simulink model "punto3"  (R2017b)
settings: Solver=VariableStepAuto  StartTime=0.0  StopTime=.3  RelTol=1e-3
values from neighbouring files (symbols this model uses):
  T0 = 0.015    [Practica2Control3.m]
  Tcarga = 0.15    [Practica2Control3.m]
  Va = 100    [Practica2Control3.m]
undefined symbols (not defined in the file or in its folder): d1c, d1d, d2d, n1c, n1d, n2c, n2d
settings Model: Creator=Agustin  LastModifiedBy=Agustin

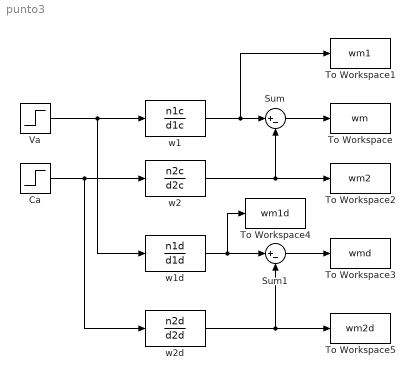
== system punto3 ==
  Ca : Step  Time=Tcarga  SampleTime=0
  Sum : Sum  Inputs=|+-
  Sum1 : Sum  Inputs=|+-
  To Workspace : ToWorkspace  VariableName=wm  SaveFormat=Timeseries  SampleTime=-1
  To Workspace1 : ToWorkspace  VariableName=wm1  SaveFormat=Timeseries  SampleTime=-1
  To Workspace2 : ToWorkspace  VariableName=wm2  SaveFormat=Timeseries  SampleTime=-1
  To Workspace3 : ToWorkspace  VariableName=wmd  SaveFormat=Timeseries  SampleTime=-1
  To Workspace4 : ToWorkspace  VariableName=wm1d  SaveFormat=Timeseries  SampleTime=-1
  To Workspace5 : ToWorkspace  VariableName=wm2d  SaveFormat=Timeseries  SampleTime=-1
  Va : Step  Time=0  After=Va  SampleTime=0
  w1 : TransferFcn  Numerator=n1c  Denominator=d1c
  w1d : DiscreteTransferFcn  Numerator=n1d  Denominator=d1d  SampleTime=T0
  w2 : TransferFcn  Numerator=n2c  Denominator=d2c
  w2d : DiscreteTransferFcn  Numerator=n2d  Denominator=d2d  SampleTime=T0
  wires:
  w1/1 -> To Workspace1/1, Sum/1
  w2/1 -> To Workspace2/1, Sum/2
  Sum/1 -> To Workspace/1
  Ca/1 -> w2d/1, w2/1
  Va/1 -> w1d/1, w1/1
  w2d/1 -> Sum1/2, To Workspace5/1
  w1d/1 -> To Workspace4/1, Sum1/1
  Sum1/1 -> To Workspace3/1
